simulink model "buck_load_transient_testbench"  (R2024b)
settings: Solver=ode4  StartTime=0.0  StopTime=0.024  FixedStep=5e-7  RelTol=1e-3
settings Model: Creator=ww  LastModifiedBy=ww

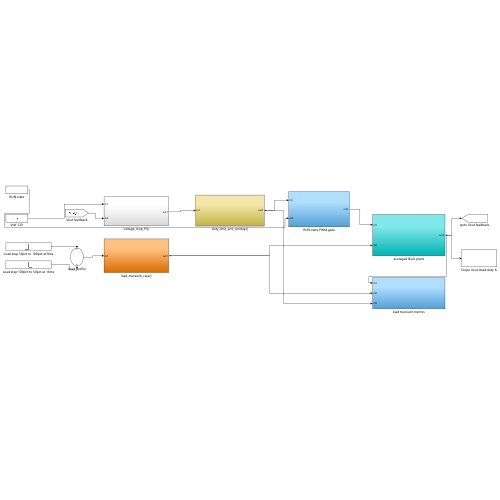
[thumbnail: Simulink's stored preview of the top-level diagram]
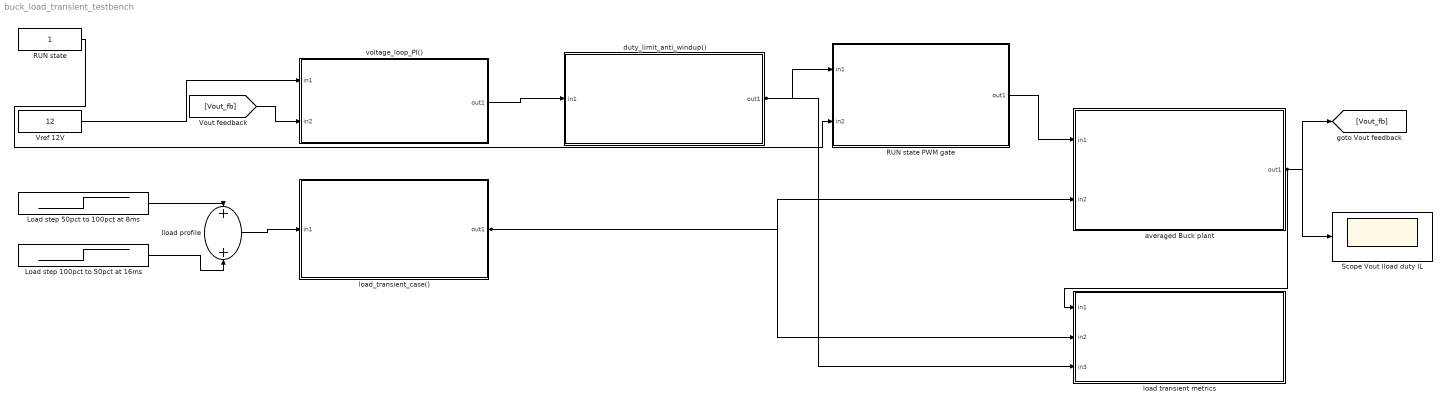
== system buck_load_transient_testbench ==
  Iload profile : Sum
  Load step 100pct to 50pct at 16ms : Step  Time=0.016  After=-2.5  SampleTime=0
  Load step 50pct to 100pct at 8ms : Step  Time=0.008  Before=2.5  After=5  SampleTime=0
  RUN state : Constant
  RUN state PWM gate : Subsystem
  Scope Vout Iload duty IL : Scope
  Vref 12V : Constant  Value=12
  averaged Buck plant : Subsystem
  duty_limit_anti_windup() : Subsystem
  load transient metrics : Subsystem
  load_transient_case() : Subsystem
  voltage_loop_PI() : Subsystem
  wires:
  Load step 50pct to 100pct at 8ms/1 -> Iload profile/1
  Load step 100pct to 50pct at 16ms/1 -> Iload profile/2
  Iload profile/1 -> load_transient_case()/1(in1)
  Vref 12V/1 -> voltage_loop_PI()/1(in1)
  [Vout_fb] -> voltage_loop_PI()/2(in2)
  voltage_loop_PI()/1(out1) -> duty_limit_anti_windup()/1(in1)
  duty_limit_anti_windup()/1(out1) -> RUN state PWM gate/1(in1), load transient metrics/3(in3)
  RUN state/1 -> RUN state PWM gate/2(in2)
  RUN state PWM gate/1(out1) -> averaged Buck plant/1(in1)
  load_transient_case()/1(out1) -> averaged Buck plant/2(in2), load transient metrics/2(in2)
  averaged Buck plant/1(out1) -> [Vout_fb], load transient metrics/1(in1), Scope Vout Iload duty IL/1

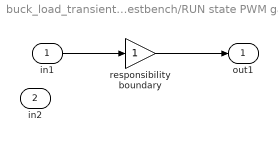
== system buck_load_transient_testbench/RUN state PWM gate ==
  in1 : Inport
  in2 : Inport  Port=2
  responsibility boundary : Gain  Description=|
      | RUN: pass duty
      | Fault or idle: duty = 0
      | This chapter keeps state in RUN
      | Protection was covered in chapter 7
  out1 : Outport
  wires:
  in1/1 -> responsibility boundary/1
  responsibility boundary/1 -> out1/1

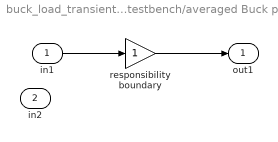
== system buck_load_transient_testbench/averaged Buck plant ==
  in1 : Inport
  in2 : Inport  Port=2
  responsibility boundary : Gain  Description=|
      | Vin = 24V
      | L = 22uH
      | C = 100uF
      | Rload changes with step
      | Outputs: Vout, IL, cap current
  out1 : Outport
  wires:
  in1/1 -> responsibility boundary/1
  responsibility boundary/1 -> out1/1

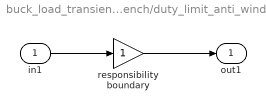
== system buck_load_transient_testbench/duty_limit_anti_windup() ==
  in1 : Inport
  responsibility boundary : Gain  Description=|
      | Clamp duty command
      | Keep raw duty observable
      | Hold integrator when saturated
      | Output: duty_cmd and saturation
  out1 : Outport
  wires:
  responsibility boundary/1 -> out1/1
  in1/1 -> responsibility boundary/1

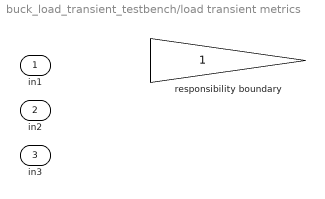
== system buck_load_transient_testbench/load transient metrics ==
  in1 : Inport
  in2 : Inport  Port=2
  in3 : Inport  Port=3
  responsibility boundary : Gain  Description=|
      | Vout undershoot
      | Vout overshoot
      | 1 percent recovery time
      | duty saturation time
      | peak inductor current

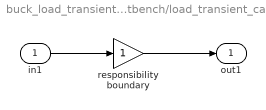
== system buck_load_transient_testbench/load_transient_case() ==
  in1 : Inport
  responsibility boundary : Gain  Description=|
      | Light load: 2.5A
      | Heavy load: 5A
      | Step up at 8ms
      | Step down at 16ms
      | Output: Rload(t) or Iload(t)
  out1 : Outport
  wires:
  responsibility boundary/1 -> out1/1
  in1/1 -> responsibility boundary/1

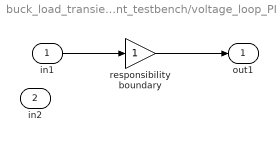
== system buck_load_transient_testbench/voltage_loop_PI() ==
  in1 : Inport
  in2 : Inport  Port=2
  responsibility boundary : Gain  Description=|
      | Input: Vref and Vout
      | Kp = 0.02
      | Ki = 80
      | Output: raw duty request
  out1 : Outport
  wires:
  in1/1 -> responsibility boundary/1
  responsibility boundary/1 -> out1/1
